simulink model "MRAS4_3"  (R2015b)
settings: Solver=ode23tb  StartTime=0.0  StopTime=0.2  MaxStep=1e-5  RelTol=1e-4
libraries: powerlib x8, powerlib_meascontrol x2, simulink x1
settings Model: Creator=Алексей  LastModifiedBy=Алексей
settings SolverCC: ZeroCrossControl=DisableAll  ZeroCrossAlgorithm=Adaptive
settings DataIOCC: LimitDataPoints=off  SaveFormat=Array  SaveOutput=off  DSMLogging=off  SaveTime=off
settings DebuggingCC: UnderspecifiedInitializationDetection=Classic  MergeDetectMultiDrivingBlocksExec=none  SolverPrmCheckMsg=warning
settings HardwareCC: ProdBitPerPointer=32  ProdLargestAtomicFloat=None  ProdIntDivRoundTo=Undefined  ProdEndianess=Unspecified  ProdWordSize=32  ProdHWDeviceType=32-bit Generic
settings GRTTargetCC: GeneratePreprocessorConditionals=Disable all
settings ConfigComp: CovModelRefEnable=Off  CovSFcnEnable=off

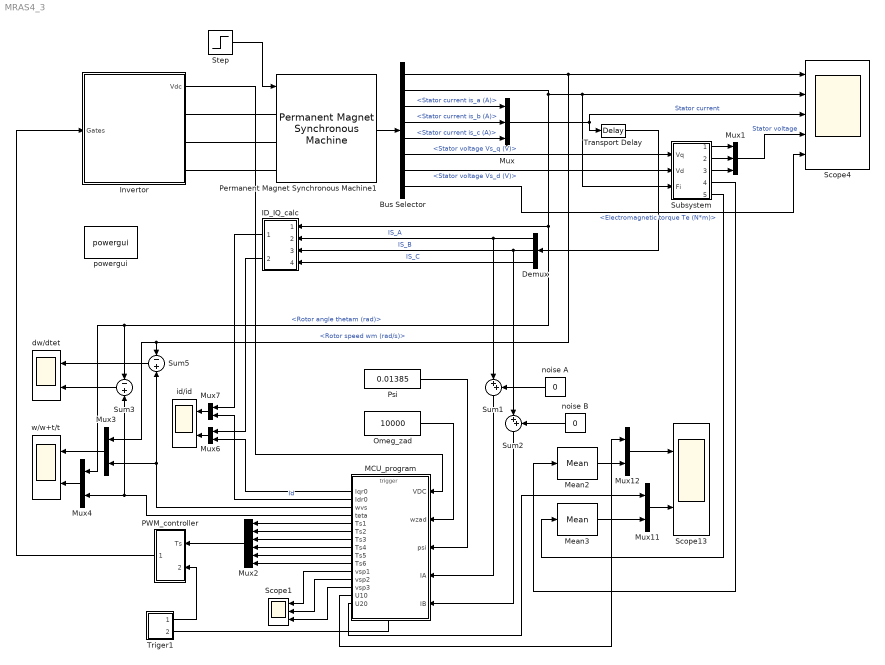
== system MRAS4_3 ==
  Bus Selector : BusSelector  OutputSignals=Rotor speed wm (rad/s),Rotor angle thetam (rad),Stator current is_a (A),Stator current is_b (A),Stator current is_c (A),Stator voltage Vs_q (V),Stator voltage Vs_d (V),Electromagnetic torque Te (N*m)
  Demux : Demux  Outputs=3
  ID_IQ_calc : Subsystem
  Invertor : Subsystem
  MCU_program : MATLAB Function  TreatAsAtomicUnit=on
  Mean2 : powerlib_meascontrol/Measurements/Mean  Freq=20000  Vinit=0  Ts=0
  Mean3 : powerlib_meascontrol/Measurements/Mean  Freq=20000  Vinit=0  Ts=0
  Mux : Mux  Inputs=3
  Mux1 : Mux  Inputs=3
  Mux{3..4,6..7,11..12} (6 alike) : Mux  Inputs=2
  Mux2 : Mux  Inputs=6
  Omeg_zad : Constant  Value=10000
  PWM_controller : Subsystem
  Permanent Magnet Synchronous Machine1 : powerlib/Machines/Permanent Magnet Synchronous Machine  NbPhases=3  FluxDistribution=Sinusoidal  RotorType=Round  MechanicalLoad=Torque Tm  PresetModel=No  ShowDetailedParameters=on  MeasurementBus=off  Resistance=0.4  Inductance=8.5e-3  dqInductances=[8.5e-3,8.5e-3]  La=294e-06  MachineConstant=Flux linkage established by magnets (V.s)  Flux=0.01385  VoltageCst=2.5121  TorqueCst=0.020775  Flat=120  Mechanical=[2e-05 1e-06 1 0]  PolePairs=1  InitialConditions=[0,0, 0,0]  InitialConditions5ph=[0 0 0 0 0 0]  TsPowergui=0  TsBlock=-1  RefAngle=Aligned with phase A axis (original Park)
  Psi : Constant  Value=0.01385
  Scope1 : Scope  NumInputPorts=3
  Scope13 : Scope  NumInputPorts=2
  Scope4 : Scope  NumInputPorts=5
  Step : Step  Time=0.5  Before=0.01  After=0.07  SampleTime=0
  Subsystem : Subsystem
  Sum1 : Sum  Inputs=|++
  Sum2 : Sum  Inputs=|++
  Sum3 : Sum  Inputs=-+
  Sum5 : Sum  Inputs=-+
  Transport Delay : TransportDelay  DelayTime=5e-6
  Triger1 : Subsystem
  dw/dtet : Scope  NumInputPorts=2
  id/id : Scope  NumInputPorts=2
  noise A : Constant  Value=0
  noise B : Constant  Value=0
  powergui : powerlib/powergui  Priority=1  SimulationMode=Continuous  SolverType=Tustin  SampleTime=50e-6  frequency=60  SPID=off  DisableSnubberDevices=off  DisableRonSwitches=off  DisableVfSwitches=off  SwTol=0  DisplayEquations=off  Interpol=off  ExternalGateDelay=off  methode=off  Ts=0  FunctionMessages=off  echomessages=off  HookPort=off  EnableUseOfTLC=off  x0status=blocks  frequencyindice=0  Pbase=100e6  ErrMax=1e-4  Iterations=50  UnitsV=kV  UnitsW=MW  buscounter=0  RestoreLinks=warning  ResistiveCurrentMeasurement=off  Frange=[0:2:500]  Ylog=off  Xlog=on  ShowGrid=off  save=off  variable=ZData  structure=SD2  ZoomFFT=on  StartTime=0.7  cycles=10  DisplayStyle=4  fundamental=382  FreqAxis=off  MaxFrequency=50000  frequencyindicesteady=1  RmsSteady=1  display=off
  w/w+t/t : Scope  NumInputPorts=2
  wires:
  Demux/1 -> ID_IQ_calc/2(In2), Sum1/1  "IS_A"
  Demux/2 -> ID_IQ_calc/3(In3), Sum2/1  "IS_B"
  MCU_program/2(Idr0) -> Mux7/2  "Id"
  Omeg_zad/1 -> MCU_program/2(wzad)
  Permanent Magnet Synchronous Machine1/1 -> Bus Selector/1
  Bus Selector/3 -> Mux/1  "<Stator current is_a (A)>"
  Bus Selector/4 -> Mux/2  "<Stator current is_b (A)>"
  Bus Selector/5 -> Mux/3  "<Stator current is_c (A)>"
  Bus Selector/6 -> Subsystem/1(Vq)  "<Stator voltage Vs_q (V)>"
  Bus Selector/7 -> Subsystem/2(Vd)  "<Stator voltage Vs_d (V)>"
  Subsystem/2(Out2) -> Mux1/2
  Subsystem/3(Out3) -> Mux1/3
  Subsystem/1(Out1) -> Mux1/1
  Mux/1 -> Scope4/3, Transport Delay/1  "Stator current"
  MCU_program/3(wvs) -> Mux3/2, Sum5/2
  Mux1/1 -> Scope4/4  "Stator voltage"
  Bus Selector/8 -> Scope4/5  "<Electromagnetic torque Te (N*m)>"
  Mux7/1 -> id/id/1
  Mux6/1 -> id/id/2
  Demux/3 -> ID_IQ_calc/4(In4)  "IS_C"
  Sum3/1 -> dw/dtet/2
  Sum5/1 -> dw/dtet/1
  MCU_program/4(teta) -> Mux4/2, Sum3/2
  ID_IQ_calc/1(Out1) -> Mux7/1
  ID_IQ_calc/2(Out2) -> Mux6/1
  Step/1 -> Permanent Magnet Synchronous Machine1/1
  MCU_program/5(Ts1) -> Mux2/1
  MCU_program/6(Ts2) -> Mux2/2
  MCU_program/7(Ts3) -> Mux2/3
  MCU_program/8(Ts4) -> Mux2/4
  MCU_program/9(Ts5) -> Mux2/5
  MCU_program/10(Ts6) -> Mux2/6
  Mux2/1 -> PWM_controller/1(Ts)
  Triger1/1(1) -> PWM_controller/2(pila)
  PWM_controller/1(Tss) -> Invertor/1(Gates)
  Mux3/1 -> w/w+t/t/1
  Mux4/1 -> w/w+t/t/2
  MCU_program/12(vsp2) -> Scope1/2
  MCU_program/13(vsp3) -> Scope1/3
  MCU_program/11(vsp1) -> Scope1/1
  Sum1/1 -> MCU_program/4(IA)
  Sum2/1 -> MCU_program/5(IB)
  Psi/1 -> MCU_program/3(psi)
  MCU_program/14(U10) -> Mux12/1
  Bus Selector/1 -> Scope4/1, Mux3/1, Sum5/1  "<Rotor speed wm (rad/s)>"
  Bus Selector/2 -> Mux4/1, Sum3/1, ID_IQ_calc/1(In1), Scope4/2, Subsystem/3(Fi)  "<Rotor angle thetam (rad)>"
  Triger1/2(2) -> MCU_program/Trigger
  MCU_program/15(U20) -> Mux11/1
  Mux12/1 -> Scope13/1
  Mux11/1 -> Scope13/2
  Mean3/1 -> Mux11/2
  Mean2/1 -> Mux12/2
  Invertor/1(Vdc) -> MCU_program/1(VDC)
  Subsystem/4(Out4) -> Mean2/1
  Subsystem/5(Out5) -> Mean3/1
  Transport Delay/1 -> Demux/1
  MCU_program/1(Iqr0) -> Mux6/2
  noise A/1 -> Sum1/2
  noise B/1 -> Sum2/2
  connections:
  Permanent Magnet Synchronous Machine1/LConn1 -- Invertor/RConn1
  Invertor/RConn3 -- Permanent Magnet Synchronous Machine1/LConn3
  Permanent Magnet Synchronous Machine1/LConn2 -- Invertor/RConn2

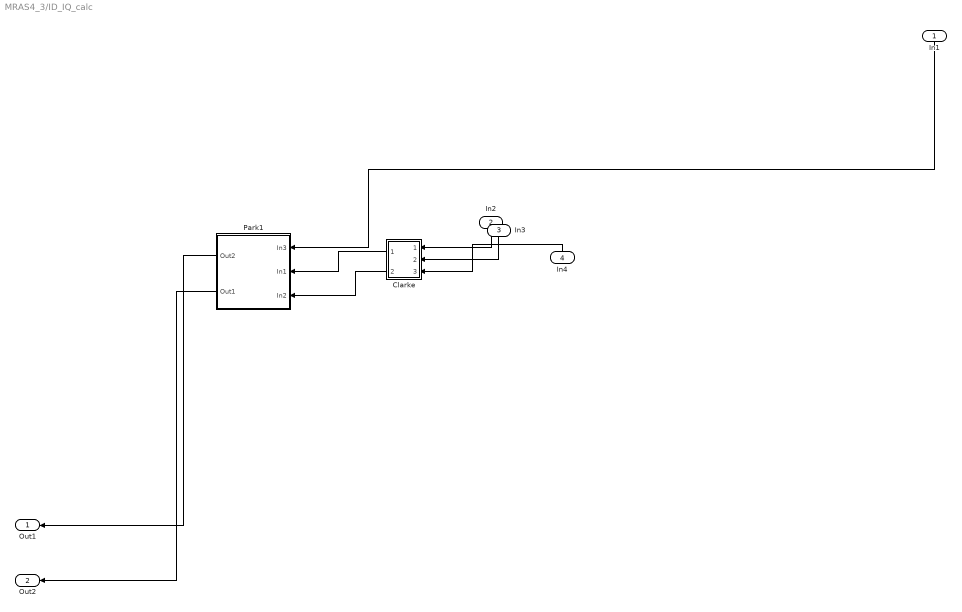
== system MRAS4_3/ID_IQ_calc ==
  In1 : Inport
  In2 : Inport  Port=2
  In3 : Inport  Port=3
  In4 : Inport  Port=4
  Clarke : Subsystem
  Park1 : Subsystem
  Out1 : Outport
  Out2 : Outport  Port=2
  wires:
  Park1/2(Out1) -> Out2/1
  Clarke/2(Out1) -> Park1/3(In2)
  Park1/1(Out2) -> Out1/1
  Clarke/1(Out2) -> Park1/2(In1)
  In1/1 -> Park1/1(In3)
  In4/1 -> Clarke/3(In3)
  In2/1 -> Clarke/1(In1)
  In3/1 -> Clarke/2(In2)

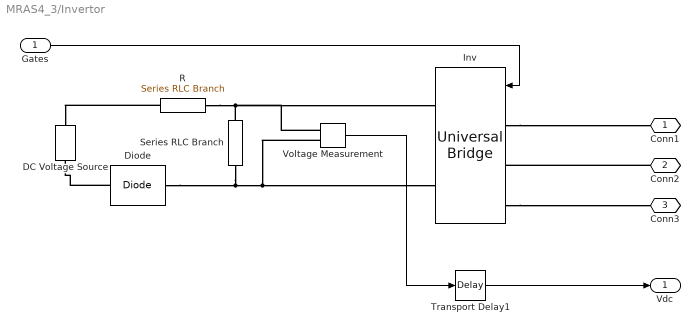
== system MRAS4_3/Invertor ==
  Gates : Inport
  DC Voltage Source : powerlib/Electrical Sources/DC Voltage Source  Amplitude=310  Measurements=None
  Diode : powerlib/Power Electronics/Diode  Ron=0.001  Lon=0  Vf=0.8  IC=0  UseSnubber=off  Rs=500  Cs=250e-9  Measurements=off
  Inv : powerlib/Power Electronics/Universal Bridge  Arms=3  SnubberResistance=1e5  SnubberCapacitance=inf  Device=IGBT / Diodes  Ron=1e-3  Lon=0  ForwardVoltages="[  0  0  ]"  ForwardVoltage=0  GTOparameters=[ 10e-6 , 20e-6 ]  IGBTparameters=[ 1e-7 , 2e-7 ]  Measurements=UAB UBC UCA UDC voltages  Measurements_2=None  converterType=Rectifier
  R : powerlib/Elements/Series RLC Branch  LConnTagsString=__new0  RConnTagsString=__new0  BranchType=R  Resistance=0.01  Inductance=1e-3  SetiL0=off  InitialCurrent=0  Capacitance=30e-6  Setx0=on  InitialVoltage=220  Measurements=None
  Series RLC Branch : powerlib/Elements/Series RLC Branch  LConnTagsString=__new0  RConnTagsString=__new0  BranchType=C  Resistance=1  Inductance=1e-3  SetiL0=off  InitialCurrent=0  Capacitance=30e-6  Setx0=on  InitialVoltage=20  Measurements=None
  Transport Delay1 : TransportDelay  DelayTime=26e-6
  Voltage Measurement : powerlib/Measurements/Voltage Measurement  PhasorSimulation=off  OutputType=Complex  PSBequivalent=0
  Conn1 : PMIOPort  Port=1  Side=Right
  Conn2 : PMIOPort  Port=2  Side=Right
  Conn3 : PMIOPort  Port=3  Side=Right
  Vdc : Outport
  wires:
  Gates/1 -> Inv/1
  Voltage Measurement/1 -> Transport Delay1/1
  Transport Delay1/1 -> Vdc/1
  connections:
  Diode/LConn1 -- Series RLC Branch/RConn1 -- Voltage Measurement/LConn2 -- Inv/RConn2
  Series RLC Branch/LConn1 -- Voltage Measurement/LConn1 -- Inv/RConn1 -- R/LConn1
  Conn2/RConn1 -- Inv/LConn2
  Diode/RConn1 -- DC Voltage Source/LConn1
  Inv/LConn3 -- Conn3/RConn1
  Inv/LConn1 -- Conn1/RConn1
  R/RConn1 -- DC Voltage Source/RConn1

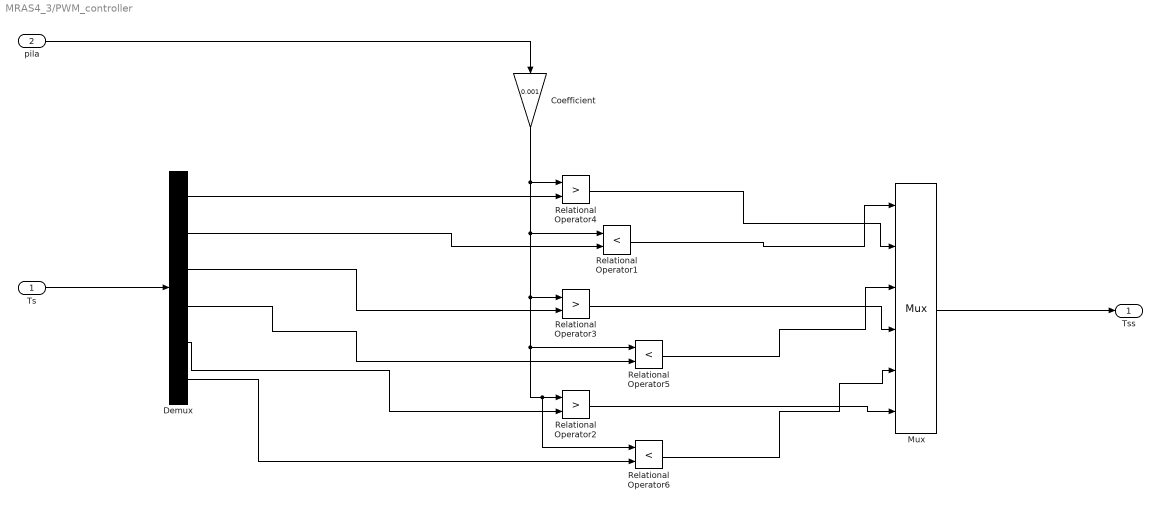
== system MRAS4_3/PWM_controller ==
  Ts : Inport
  pila : Inport  Port=2
  Coefficient : Gain  Gain=0.001
  Demux : Demux  Outputs=6
  Mux : Mux  Inputs=6
  Relational Operator1 : RelationalOperator  Operator=<  OutDataTypeStr=boolean
  Relational Operator2 : RelationalOperator  Operator=>  OutDataTypeStr=boolean
  Relational Operator3 : RelationalOperator  Operator=>  OutDataTypeStr=boolean
  Relational Operator4 : RelationalOperator  Operator=>  OutDataTypeStr=boolean
  Relational Operator5 : RelationalOperator  Operator=<  OutDataTypeStr=boolean
  Relational Operator6 : RelationalOperator  Operator=<  OutDataTypeStr=boolean
  Tss : Outport
  wires:
  Relational Operator4/1 -> Mux/2
  Demux/3 -> Relational Operator3/2
  Demux/5 -> Relational Operator2/2
  Relational Operator3/1 -> Mux/4
  Relational Operator2/1 -> Mux/6
  Ts/1 -> Demux/1
  Coefficient/1 -> Relational Operator1/1, Relational Operator3/1, Relational Operator5/1, Relational Operator6/1, Relational Operator2/1, Relational Operator4/1
  Relational Operator1/1 -> Mux/1
  Relational Operator5/1 -> Mux/3
  Relational Operator6/1 -> Mux/5
  Demux/2 -> Relational Operator1/2
  Demux/4 -> Relational Operator5/2
  Demux/6 -> Relational Operator6/2
  Demux/1 -> Relational Operator4/2
  pila/1 -> Coefficient/1
  Mux/1 -> Tss/1

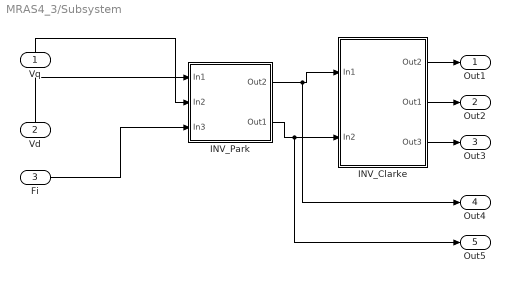
== system MRAS4_3/Subsystem ==
  Vq : Inport
  Vd : Inport  Port=2
  Fi : Inport  Port=3
  INV_Clarke : Subsystem
  INV_Park : Subsystem
  Out1 : Outport
  Out2 : Outport  Port=2
  Out3 : Outport  Port=3
  Out4 : Outport  Port=4
  Out5 : Outport  Port=5
  wires:
  INV_Clarke/2(Out1) -> Out2/1
  INV_Park/1(Out2) -> Out4/1, INV_Clarke/1(In1)
  INV_Clarke/1(Out2) -> Out1/1
  INV_Park/2(Out1) -> Out5/1, INV_Clarke/2(In2)
  INV_Clarke/3(Out3) -> Out3/1
  Fi/1 -> INV_Park/3(In3)
  Vd/1 -> INV_Park/1(In1)
  Vq/1 -> INV_Park/2(In2)

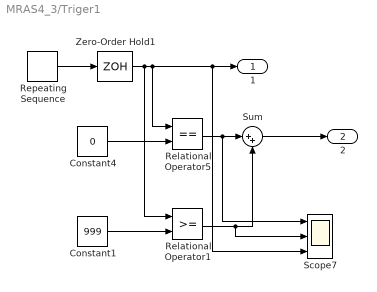
== system MRAS4_3/Triger1 ==
  Constant1 : Constant  Value=999
  Constant4 : Constant  Value=0
  Relational Operator1 : RelationalOperator  OutDataTypeStr=boolean
  Relational Operator5 : RelationalOperator  Operator===  OutDataTypeStr=boolean
  Repeating Sequence : simulink/Sources/Repeating Sequence  rep_seq_t=[0 2.5e-5 5e-5]  rep_seq_y=[0 1000 0]
  Scope7 : Scope  NumInputPorts=3
  Sum : Sum  Inputs=|++
  Zero-Order Hold1 : ZeroOrderHold  SampleTime=1e-8
  1 : Outport
  2 : Outport  Port=2
  wires:
  Zero-Order Hold1/1 -> Relational Operator1/1, Relational Operator5/1, Scope7/3, 1/1
  Repeating Sequence/1 -> Zero-Order Hold1/1
  Constant4/1 -> Relational Operator5/2
  Sum/1 -> 2/1
  Constant1/1 -> Relational Operator1/2
  Relational Operator5/1 -> Scope7/1, Sum/1
  Relational Operator1/1 -> Scope7/2, Sum/2

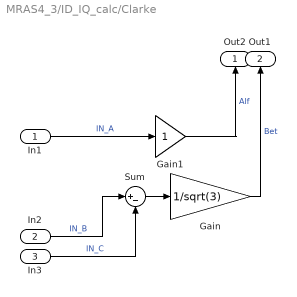
== system MRAS4_3/ID_IQ_calc/Clarke ==
  In1 : Inport
  In2 : Inport  Port=2
  In3 : Inport  Port=3
  Gain : Gain  Gain=1/sqrt(3)
  Gain1 : Gain
  Sum : Sum  Inputs=|+-
  Out2 : Outport
  Out1 : Outport  Port=2
  wires:
  Gain/1 -> Out1/1  "Bet"
  In2/1 -> Sum/1  "IN_B"
  In1/1 -> Gain1/1  "IN_A"
  In3/1 -> Sum/2  "IN_C"
  Sum/1 -> Gain/1
  Gain1/1 -> Out2/1  "Alf"

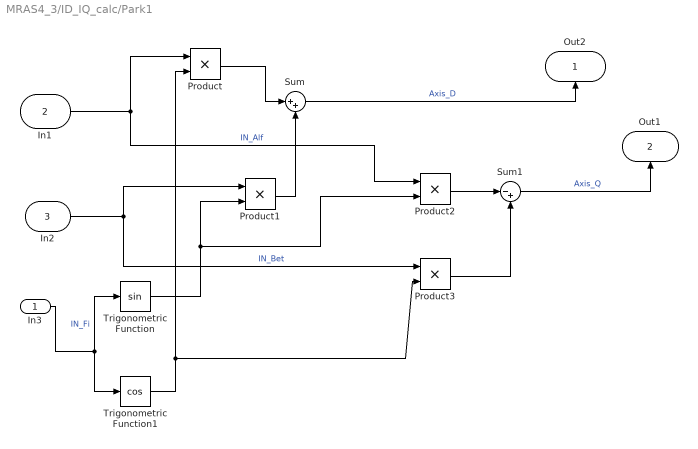
== system MRAS4_3/ID_IQ_calc/Park1 ==
  In3 : Inport
  In1 : Inport  Port=2
  In2 : Inport  Port=3
  Product{,1..3} (4 alike) : Product
  Sum : Sum  Inputs=|++
  Sum1 : Sum  Inputs=|-+
  Trigonometric Function : Trigonometry
  Trigonometric Function1 : Trigonometry  Operator=cos
  Out2 : Outport
  Out1 : Outport  Port=2
  wires:
  Sum1/1 -> Out1/1  "Axis_Q"
  In2/1 -> Product1/1, Product3/1  "IN_Bet"
  In1/1 -> Product2/1, Product/1  "IN_Alf"
  Sum/1 -> Out2/1  "Axis_D"
  In3/1 -> Trigonometric Function1/1, Trigonometric Function/1  "IN_Fi"
  Trigonometric Function1/1 -> Product/2, Product3/2
  Trigonometric Function/1 -> Product2/2, Product1/2
  Product1/1 -> Sum/2
  Product/1 -> Sum/1
  Product2/1 -> Sum1/1
  Product3/1 -> Sum1/2

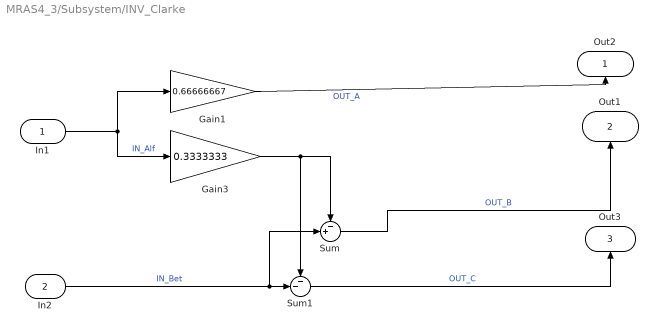
== system MRAS4_3/Subsystem/INV_Clarke ==
  In1 : Inport
  In2 : Inport  Port=2
  Gain1 : Gain  Gain=0.66666667
  Gain3 : Gain  Gain=0.3333333
  Sum : Sum  Inputs=-+|
  Sum1 : Sum  Inputs=--|
  Out2 : Outport
  Out1 : Outport  Port=2
  Out3 : Outport  Port=3
  wires:
  Sum/1 -> Out1/1  "OUT_B"
  In2/1 -> Sum/2, Sum1/2  "IN_Bet"
  In1/1 -> Gain1/1, Gain3/1  "IN_Alf"
  Gain1/1 -> Out2/1  "OUT_A"
  Sum1/1 -> Out3/1  "OUT_C"
  Gain3/1 -> Sum1/1, Sum/1

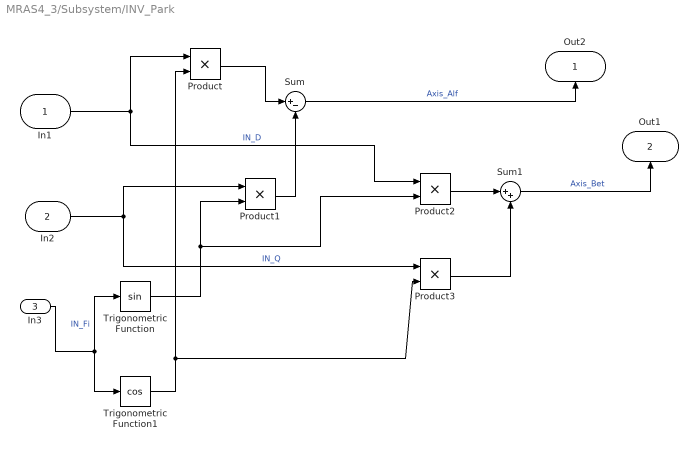
== system MRAS4_3/Subsystem/INV_Park ==
  In1 : Inport
  In2 : Inport  Port=2
  In3 : Inport  Port=3
  Product{,1..3} (4 alike) : Product
  Sum : Sum  Inputs=|+-
  Sum1 : Sum  Inputs=|++
  Trigonometric Function : Trigonometry
  Trigonometric Function1 : Trigonometry  Operator=cos
  Out2 : Outport
  Out1 : Outport  Port=2
  wires:
  Sum1/1 -> Out1/1  "Axis_Bet"
  In2/1 -> Product1/1, Product3/1  "IN_Q"
  In1/1 -> Product2/1, Product/1  "IN_D"
  Sum/1 -> Out2/1  "Axis_Alf"
  In3/1 -> Trigonometric Function1/1, Trigonometric Function/1  "IN_Fi"
  Trigonometric Function1/1 -> Product/2, Product3/2
  Trigonometric Function/1 -> Product2/2, Product1/2
  Product1/1 -> Sum/2
  Product/1 -> Sum/1
  Product2/1 -> Sum1/1
  Product3/1 -> Sum1/2

== matlab function MRAS4_3/MCU_program ==
  data: Iqr0 output; VDC input; wzad input; Idr0 output; psi input; wvs output; teta output; IA input; IB input; Ts1 output; Ts2 output; Ts3 output; Ts4 output; Ts5 output; Ts6 output; vsp1 output; vsp2 output; vsp3 output; U10 output; U20 output
  events: trigger input RISING_EDGE_EVENT
function [Iqr0,Idr0,wvs,teta,Ts1,Ts2,Ts3,Ts4,Ts5,Ts6,vsp1,vsp2,vsp3,U10,U20] = fcn(VDC,wzad,psi,IA,IB)
R=0.35;
L=294e-6;

cur_lim=10;

dt=25e-6;
kint=1000;
kp=0.16;
Idzad=0;

wstart=150;

eps=1500;

ktp=0.001;
kti=0.075;

kuqp=2;
kuqi=2;

kudp=2;
kudi=2;

persistent wrez1;
persistent tet1;
persistent Idr1;
persistent Iqr1;
persistent count1;
persistent Ialfa;
persistent Ibeta;
persistent wrez;
persistent omeg;
persistent count_om;
persistent tew;
persistent tet;
persistent wint;
persistent dId;
persistent dIq;
persistent Id; 
persistent Iq;
persistent Ua0; 
persistent Ub0;
persistent count;
persistent torque_int;
persistent voltageq_int;
persistent voltaged_int;

persistent phase;
persistent wst;
persistent phase1;
persistent vmodi_int;
persistent fl;

persistent id_lim;
persistent iq_lim;
persistent cur_lim_fl;
persistent cur_lim_fl2;


persistent w_fl;


%заполнение начальных значений static переменным (persistent здесь)
if isempty(wrez1)
    wrez1=0;
end 

if isempty(tet1)
    tet1=0;
end 
if isempty(Idr1)
    Idr1=0;
end 

if isempty(Iqr1)
    Iqr1=0;
end 
if isempty(count1)
    count1=0;
end 


if isempty(wrez)
    wrez=0;
end 

if isempty(omeg)
    omeg=0;
end 

if isempty(count_om)
    count_om=0;
end 

if isempty(tew)
    tew=0;
end 

if isempty(tet)
    tet=0;
end 

if isempty(wint)
    wint=0;
end 

if isempty(Ua0)
    Ua0=0;
end   
if isempty(Ub0)
    Ub0=0;
end

if isempty(Id)
    Id=0;
end   
if isempty(Iq)
    Iq=0;
end
if isempty(count)
    count=0;
end
if isempty(torque_int)
    torque_int=0;
end 

if isempty(voltageq_int)
    voltageq_int=0;
end 

if isempty(voltaged_int)
    voltaged_int=0;
end 

if isempty(wst)
    wst=0;
end 
if isempty(phase1)
    phase1=0;
end 

if isempty(vmodi_int)
    vmodi_int=0;
end 
if isempty(fl)
    fl=0;
end 
if isempty(id_lim)
    id_lim=0;
end 

if isempty(iq_lim)
    iq_lim=0;
end 

if isempty(cur_lim_fl)
    cur_lim_fl=0;
end 
if isempty(cur_lim_fl2)
    cur_lim_fl2=0;
end 

if isempty(w_fl)
    w_fl=0;
end 

%Кларк

Ialfa=IA;
Ibeta=(2*IB+IA)/1.7320508;


%Расчёт напряжений по осям Дэ и Ку  (парк)
Ud=Ua0*cos(tet+wrez*dt/2)+Ub0*sin(tet+wrez*dt/2);                           %15.11 добавлено +wrez*dt/2
Uq=Ub0*cos(tet+wrez*dt/2)-Ua0*sin(tet+wrez*dt/2);                           %15/11 добавлено +wrez*dt/2

% производные нового шага для рассчётных значений токов Id и Iq
dId=-R/L*Id+wrez*Iq+Ud/L;
dIq=-wrez*Id-R/L*Iq-wrez*psi/L+Uq/L;


%рассчётные значения токов Id и Iq через производные 
Id=Id+dId*dt;
Iq=Iq+dIq*dt;


    
%реальные значения токов Id и Iq, полученные через  угол и оси альфа,бета 
Idr=Ialfa*cos(tet)+Ibeta*sin(tet);
Iqr=Ibeta*cos(tet)-Ialfa*sin(tet); 

%производная скорости через МРАС
dw=Idr*Iq-Id*Iqr-(Iqr-Iq)*psi/L;


%ПИ-регулятор
        %интегральная составляющая

wint=wint+kint*dw*dt;
        %пропорциональная составляющая
wp=dw*kp;
    % результирующая П и И составяющая

wrez=wint+wp;


%Определение углового положения ротора
tet=tet+wrez*dt;

%Усреднение скорости за 5 периодов для ПИ-регуляторов
%контура регулирования скорости
count1=count1+1;
if count1>4
count1=0;
omeg=tet-tew;
omeg=omeg/dt/5;
tew=tet;
end

%если скорость сильно ниже требуемой, то интегратор отключен,
%пропроциональная составляющая 0.5
if omeg>0.98*wzad
    fl=1;
end
    
    
if (fl==0)
 torque_pr=0.5;
 torque_int=0;
% если скорость приблизилась к требуемой, то стандартный ПИД алгоритм
else    
 torque_pr=(wzad-omeg)*ktp;
 
 if (abs(wzad-omeg)>15)
    torque_int=torque_int+(wzad-omeg)*kti*dt;
 end
  if torque_int>0.5
     torque_int=0.5;
  end    

     if torque_int+torque_pr>0.5
         torque_pr=0.5-torque_int;
     end
     
   if torque_int<0 
       torque_int=0; 
   end 
end


 %формирование момента, требуемого на валу   
torque=torque_pr+torque_int;

% определение поперечной составляющей тока, для требуемого момента
cur_q=torque*0.67/psi;

if (cur_q>cur_lim) 
    cur_q=cur_lim;
elseif (cur_q<0.01)
    cur_q=0.01;
end

if (cur_lim_fl==0)
    iq_lim=Iqr;
    
    if (iq_lim<0)
     iq_lim=0;
    end
    id_lim=Idr;
elseif (cur_lim_fl2==0)
    if (iq_lim<cur_q-0.15) 
      iq_lim=iq_lim+0.1;
      id_lim=sqrt(cur_lim^2-iq_lim^2);
    else
        cur_lim_fl2=1;
    end;
else
    iq_lim=cur_q;
    id_lim=Idzad;
end;



%ПИ-регулятор для напряжения по оси Ку
diq=iq_lim-Iqr;
voltageq_pr=diq*kuqp;
voltageq_int=voltageq_int+diq*kuqi*dt;

voltage_q=voltageq_pr+voltageq_int+1.5*(L*Idr+psi)*wrez;                    %15.11 поменял на omeg на wrez, интересно, как скажется на точности


%ПИ-регулятор для напряжения по оси Дэ
did=id_lim-Idr;
voltaged_pr=did*kudp;
voltaged_int=voltaged_int+did*kudi*dt;

voltage_d=voltaged_pr+voltaged_int-1.5*(wrez*Iqr*L);                        %15.11 поменял на omeg на wrez, интересно, как скажется на точности


%Согласование уровней напряжений Уд и Уку с питанием


k=0.75;                                          %коэффициент напряжения питания%


if(voltage_d)^2+(voltage_q)^2>=(k*VDC)^2         %сравнение значений результирующего вектора напряжения и напряжения источника питания%
    if abs(voltage_d)<k*VDC                      %сравнение величины модуля составляющей Ud с величиной напряжения источника питания%
    voltage_q=sqrt(((k*VDC)^2)-(voltage_d)^2);    %коррекция Uq в случае, если составляющая Ud не превышает напряжение питания%
    else
        voltage_d=-k*VDC;                        %коррекция Ud в случае превышения составляющей Ud напряжения питания%
        voltage_q=0;                             %коррекция Uq в случае превышения составляющей Ud напряжения питания%
    end 
end

valf=voltage_d*cos(tet)-voltage_q*sin(tet);             
vbet=voltage_d*sin(tet)+voltage_q*cos(tet);            



if ((wrez>=wstart)&&(w_fl==0)&&(wst>25))
    w_fl=1;
end  
  
if((w_fl==1)&&(Iqr>0))
    w_fl=2;
end

cur_lim_fl=1;    
if (w_fl<0)   
  wst=wst+eps*dt;
  if (wst>wstart) 
      wst=wstart; 
  end;
    
phase1=phase1+wst*dt;
     
% Парк
Idvs=Ialfa*cos(phase1)+Ibeta*sin(phase1);

Iqvs=Ibeta*cos(phase1)-Ialfa*sin(phase1);

  Uqvs=(cur_lim-Iqvs)*10;
  Udvs=-Idvs*10;
     
  valf=Udvs*cos(phase1)-Uqvs*sin(phase1);
  vbet=Udvs*sin(phase1)+Uqvs*cos(phase1);
  
  voltageq_int=0;
  voltaged_int=0;
    
  cur_lim_fl=0;
    
end



Ua0=valf;
Ub0=vbet;


U10=Ua0;
U20=Ub0;

vref=sqrt(valf^2+vbet^2);
phase=acos(valf/vref)*sign(vbet)+(sign(vbet)-1)*(-pi);
vrefa=vref*1.5;
vphase=phase;


%вывод на осциллографы


teta=tet;
wvs=wrez;
Idr0=Idr;
Iqr0=Iqr;

vsp1=cur_lim_fl;
vsp2=id_lim;
vsp3=iq_lim;




%алгоритм формирования векторной ШИМ  мертвым веменем dead [мкс]
dead=0.75;
dead=dead/25;
a=vphase;
v2=vrefa;
%Tz=dt/6;
if a>=0 && a<pi/3 
    n=1;
elseif  a>=pi/3 && a<2*pi/3 
    n=2;
elseif  a>=2*pi/3 && a<pi 
    n=3;
elseif  a>=pi && a<4*pi/3 
    n=4;
elseif  a>=4*pi/3 && a<5*pi/3 
    n=5;
else n=6;

end


a_cor=a-(n-1)*pi/3;

T1 = (v2/VDC)*sin(pi/3-a_cor)/sin(pi/3);
T2 = (v2/VDC)*sin(a_cor)/sin(pi/3);
T0=1-T1-T2;
Ta1=0; Ta3=0; Ta5=0; 
switch n
    case 1
        
        Ta1=T1+T2+T0/2;
        
        Ta3=T2+T0/2;
       
        Ta5=T0/2;
       
    case 2
        
        Ta1=T1+T0/2;
        
        Ta3=T1+T2+T0/2;
    
        Ta5=T0/2;       
        
    case 3
        
        Ta1=T0/2;
       
        Ta3=T1+T2+T0/2;
       
        Ta5=T2+T0/2;    
        
    case 4
        
        Ta1=T0/2;
       
        Ta3=T1+T0/2;
       
        Ta5=T1+T2+T0/2;   
       
    case 5
        
        Ta1=T2+T0/2;
        
        Ta3=T0/2;
        
        Ta5=T1+T2+T0/2;     
        
    case 6
        
        Ta1=T1+T2+T0/2;
        
        Ta3=T0/2;
     
        Ta5=T1+T0/2;    
        
end;


Ts1=(Ta1)+dead/2; 
Ts3=(Ta3)+dead/2; 
Ts5=(Ta5)+dead/2;
Ts2=(Ta1)-dead/2; 
Ts4=(Ta3)-dead/2; 
Ts6=(Ta5)-dead/2;


if (IA>0) 
    Ts1=Ts1+dead/2;
    Ts2=Ts2+dead/2;
else
    Ts1=Ts1-dead/2;
    Ts2=Ts2-dead/2;           
end;
if (IB>0) 
    Ts3=Ts3+dead/2;
    Ts4=Ts4+dead/2;
else
    Ts3=Ts3-dead/2;
    Ts4=Ts4-dead/2; 
end;  
if ((-IA-IB)>0) 
    Ts5=Ts5+dead/2;
    Ts6=Ts6+dead/2;
else
    Ts5=Ts5-dead/2;
    Ts6=Ts6-dead/2;           
end;


return;
